simulink model "ModeloCANBus1"  (R2025b)
settings: Solver=VariableStepAuto  StartTime=0.0  StopTime=10.0  RelTol=1e-3
undefined symbols (not defined in the file): canChannel
libraries: canlib x3, canmsglib x2
settings Model: Creator=usuario  LastModifiedBy=usuario

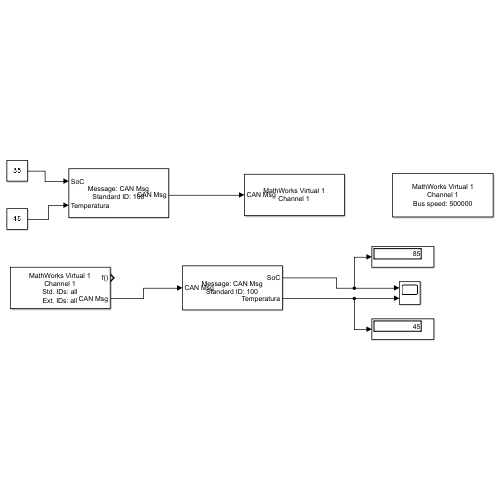
[thumbnail: Simulink's stored preview of the top-level diagram]
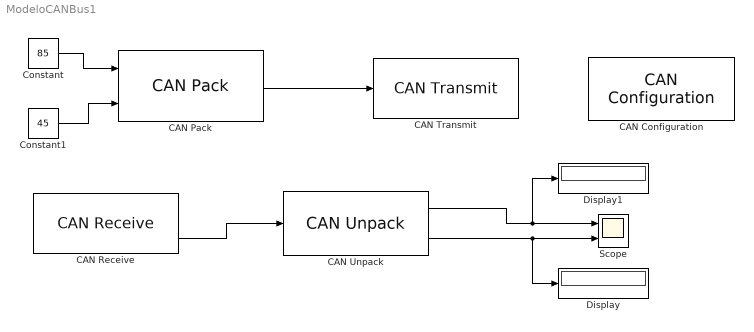
== system ModeloCANBus1 ==
  CAN Configuration : canlib/CAN Configuration  BlockHandle=157.0001  Device=MathWorks Virtual 1 (Channel 1)  DeviceMenu=MathWorks Virtual 1 (Channel 1)  ObjConstructor=canChannel('MathWorks', 'Virtual 1', 1)  BusSpeed=500000  EnableBitParameters=off  AckMode=Normal
  CAN Pack : canmsglib/CAN Pack  MsgList=(none)  MsgName=CAN Msg  MsgIDType=Standard (11-bit identifier)  MsgIdentifier=100  CANIDInput=off  MsgLength=8  Remote=off  ApplyMinMax=off  BusOutput=off  SignalInfo={ 'SoC', '0', '8', 'LE', 'signed', 'Standard', '0', '1', '0', '-Inf', 'Inf'; 'Temperatura', '8', '8', 'LE', 'signed', 'Standard', '0', '1', '0', '-Inf', 'Inf' }
      settings: LibrarySourceBlock=canlib/CAN Pack  DataFormat=manually specified signals
  CAN Receive : canlib/CAN Receive  BlockHandle=162.0001  Device=MathWorks Virtual 1 (Channel 1)  DeviceMenu=MathWorks Virtual 1 (Channel 1)  ObjConstructor=canChannel('MathWorks', 'Virtual 1', 1)  EnableStandardIDsFilter=off  StdIDsCombo=Allow all  StandardIDs=0  EnableExtendedIDsFilter=off  ExtIDsCombo=Allow all  ExtendedIDs=0  SampleTime=0.01  MsgsPerTimestep=all  InternalFilterUpdateStatus=on  BusOutput=off
  CAN Transmit : canlib/CAN Transmit  BlockHandle=166.0002  Device=MathWorks Virtual 1 (Channel 1)  DeviceMenu=MathWorks Virtual 1 (Channel 1)  ObjConstructor=canChannel('MathWorks', 'Virtual 1', 1)  EnableEventTransmit=off  EnablePeriodicTransmit=off  MessagePeriod=1.000
  CAN Unpack : canmsglib/CAN Unpack  MsgList=(none)  MsgName=CAN Msg  MsgIDType=Standard (11-bit identifier)  MsgIdentifier=100  MsgLength=8  SignalInfo={ 'SoC', '0', '8', 'LE', 'signed', 'Standard', '0', '1', '0', '-Inf', 'Inf'; 'Temperatura', '8', '8', 'LE', 'signed', 'Standard', '0', '1', '0', '-Inf', 'Inf' }  IDPort=off  TimestampPort=off  ErrorPort=off  RemotePort=off  LengthPort=off  StatusPort=off  ApplyMinMax=off
      settings: LibrarySourceBlock=canlib/CAN Unpack
  Constant : Constant  Value=85
  Constant1 : Constant  Value=45
  Display : Display
  Display1 : Display
  Scope : Scope  NumInputPorts=2
      settings: ActiveDisplayYMinimum=-10.624999999999998  ActiveDisplayYMaximum=95.625
  wires:
  Constant/1 -> CAN Pack/1
  Constant1/1 -> CAN Pack/2
  CAN Pack/1 -> CAN Transmit/1
  CAN Receive/2 -> CAN Unpack/1
  CAN Unpack/1 -> Display1/1, Scope/1
  CAN Unpack/2 -> Display/1, Scope/2
